simulink subsystem "electrical_power_subsystem"  (R2023b)
settings: Solver=VariableStepAuto  StartTime=0.0  StopTime=10.0  RelTol=1e-3
settings Model: Creator=gio  LastModifiedBy=gio

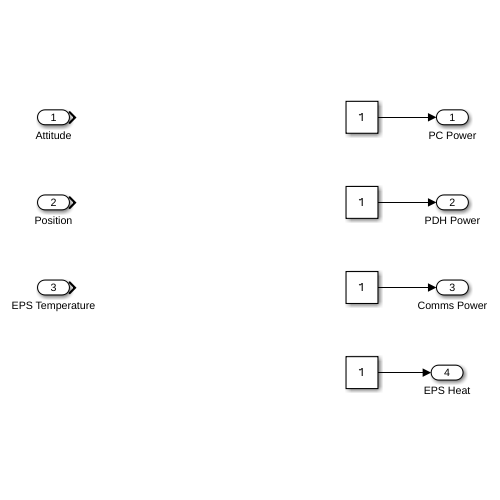
[thumbnail: Simulink's stored preview of the top-level diagram]
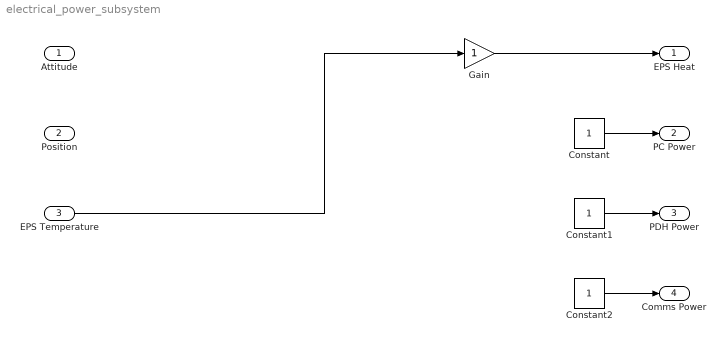
== system electrical_power_subsystem ==
  Attitude : Inport
  Position : Inport  Port=2
  EPS Temperature : Inport  Port=3
  Constant : Constant
  Constant1 : Constant
  Constant2 : Constant
  Gain : Gain
  EPS Heat : Outport
  PC Power : Outport  Port=2
  PDH Power : Outport  Port=3
  Comms Power : Outport  Port=4
  wires:
  Constant/1 -> PC Power/1
  Constant1/1 -> PDH Power/1
  Constant2/1 -> Comms Power/1
  Gain/1 -> EPS Heat/1
  EPS Temperature/1 -> Gain/1
